simulink model "CAN_communication"  (R2022a)
settings: Solver=VariableStepAuto  StartTime=0.0  StopTime=1000.0  RelTol=1e-3
undefined symbols (not defined in the file or in its folder): canChannel
libraries: canlib x3, canmsglib x2
settings Model: Creator=Haricharan Projects  LastModifiedBy=Haricharan Projects

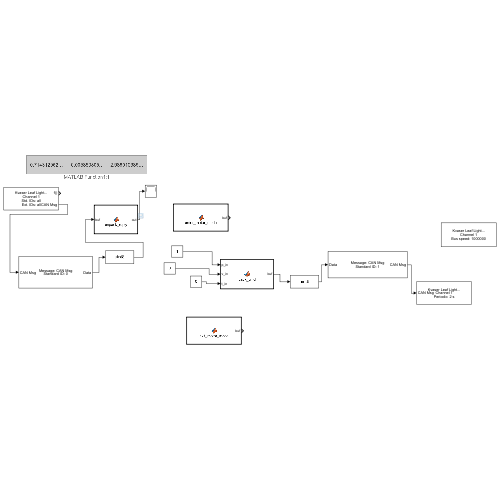
[thumbnail: Simulink's stored preview of the top-level diagram]
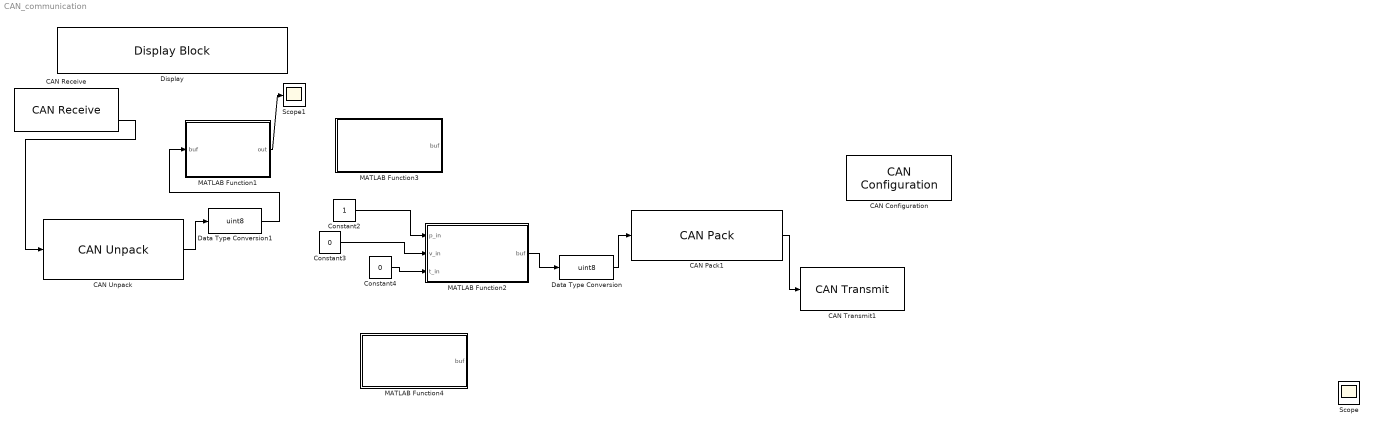
== system CAN_communication ==
  CAN Configuration : canlib/CAN Configuration  BlockHandle=12.1127  Device=MathWorks Virtual 1 (Channel 1)  DeviceMenu=MathWorks Virtual 1 (Channel 1)  ObjConstructor=canChannel('MathWorks', 'Virtual 1', 1)  BusSpeed=500000  EnableBitParameters=off  AckMode=Normal
      settings: SourceProductBaseCode=VN
  CAN Pack1 : canmsglib/CAN Pack  MsgList=(none)  MsgName=CAN Msg  MsgIDType=Standard (11-bit identifier)  MsgIdentifier=1  MsgLength=8  Remote=off  ApplyMinMax=off  BusOutput=off  SignalInfo={}
      settings: SourceProductBaseCode=XP,ME,VN  DataFormat=raw data
  CAN Receive : canlib/CAN Receive  BlockHandle=16.0028  Device=MathWorks Virtual 1 (Channel 1)  DeviceMenu=MathWorks Virtual 1 (Channel 1)  ObjConstructor=canChannel('MathWorks', 'Virtual 1', 1)  EnableStandardIDsFilter=off  StdIDsCombo=Allow all  StandardIDs=0  EnableExtendedIDsFilter=off  ExtIDsCombo=Allow all  ExtendedIDs=0  SampleTime=0.01  MsgsPerTimestep=all  InternalFilterUpdateStatus=on  BusOutput=off
      settings: SourceProductBaseCode=VN
  CAN Transmit1 : canlib/CAN Transmit  BlockHandle=19.0005  Device=MathWorks Virtual 1 (Channel 1)  DeviceMenu=MathWorks Virtual 1 (Channel 1)  ObjConstructor=canChannel('MathWorks', 'Virtual 1', 1)  EnableEventTransmit=off  EnablePeriodicTransmit=on  MessagePeriod=2.000
      settings: SourceProductBaseCode=VN
  CAN Unpack : canmsglib/CAN Unpack  MsgList=(none)  MsgName=CAN Msg  MsgIDType=Standard (11-bit identifier)  MsgIdentifier=0  MsgLength=8  SignalInfo={}  IDPort=off  TimestampPort=off  ErrorPort=off  RemotePort=off  LengthPort=off  StatusPort=off  ApplyMinMax=off
      settings: SourceProductBaseCode=XP,ME,VN  DataFormat=raw data
  Constant2 : Constant  SampleTime=2
  Constant3 : Constant  Value=0  SampleTime=2
  Constant4 : Constant  Value=0  SampleTime=2
  Data Type Conversion : DataTypeConversion  OutDataTypeStr=uint8  SaturateOnIntegerOverflow=off  RndMeth=Floor
  Data Type Conversion1 : DataTypeConversion  OutDataTypeStr=uint8  SaturateOnIntegerOverflow=off  RndMeth=Floor
  Display : DisplayBlock  LabelPosition=Bottom  Format=long  Transparency=1
  MATLAB Function1 : MATLAB Function  TreatAsAtomicUnit=on
  MATLAB Function2 : MATLAB Function  TreatAsAtomicUnit=on
  MATLAB Function3 : MATLAB Function  TreatAsAtomicUnit=on
  MATLAB Function4 : MATLAB Function  TreatAsAtomicUnit=on
  Scope1 : Scope
  Scope : Scope
  wires:
  CAN Pack1/1 -> CAN Transmit1/1
  Constant2/1 -> MATLAB Function2/1(p_in)
  Constant4/1 -> MATLAB Function2/3(t_in)
  Constant3/1 -> MATLAB Function2/2(v_in)
  CAN Receive/2 -> CAN Unpack/1
  CAN Unpack/1 -> Data Type Conversion1/1
  Data Type Conversion1/1 -> MATLAB Function1/1(buf)
  Data Type Conversion/1 -> CAN Pack1/1
  MATLAB Function1/1(out) -> Scope1/1
  MATLAB Function2/1(buf) -> Data Type Conversion/1

== matlab function CAN_communication/MATLAB Function2 ==
  data: p_in input double; buf output; v_in input; t_in input
function buf  = pack_cmd(p_in, v_in, t_in)

P_MIN = -12.5;
P_MAX = 12.5;
V_MIN = -8.0;
V_MAX = 8.0;
KP_MIN = 0.0;
KP_MAX = 500.0;
KD_MIN = 0.0;
KD_MAX = 5.0;
T_MIN = -144.0;
T_MAX = 144.0;

kp_in = 10;
kd_in = 5;

p_des = constrain(p_in, P_MIN, P_MAX);
v_des = constrain(v_in, V_MIN, V_MAX);
kp = constrain(kp_in, KP_MIN, KP_MAX);
kd = constrain(kd_in, KD_MIN, KD_MAX);
t_ff = constrain(t_in, T_MIN, T_MAX);

p_int = float_to_uint(p_des, P_MIN, P_MAX, 16);
v_int = float_to_uint(v_des, V_MIN, V_MAX, 12);
kp_int = float_to_uint(kp, KP_MIN, KP_MAX, 12);
kd_int = float_to_uint(kd, KD_MIN, KD_MAX, 12);
t_int = float_to_uint(t_ff, T_MIN, T_MAX, 12);

buf = ([0 0 0 0 0 0 0 0]);

buf(1) = bitshift(p_int, -8, 'uint64');
buf(2) = bitand(p_int, uint64(0xFF), 'uint64');
buf(3) = bitshift(v_int, -4, 'uint64');
buf(4) = bitor(bitshift(bitand(v_int, uint64(0xF), 'uint64'), +4, 'uint64'), bitshift(kp_int, -8, 'uint64'));
buf(5) = bitand(kp_int, uint64(0xFF), 'uint64');
buf(6) = bitshift(kd_int, -4, 'uint64');
buf(7) = bitor(bitshift(bitand(kd_int, uint64(0xF)), 4, 'uint64'), bitshift(t_int, -8, 'uint64'));
buf(8) = bitand(t_int, uint64(0xFF), 'uint64');

end

function [pgg] = float_to_uint(x, x_min, x_max, bits)
span = x_max - x_min;
offset = x_min;
pgg = uint64(0);

if (bits == 12)
    pgg = (x - offset) * 4095.0/ span;
    pgg = uint64(pgg);
elseif (bits == 16)
    pgg = (x - offset) * 65535.0/ span;
    pgg = uint64(pgg);
pgg = uint64(pgg);
    
end
end

function val = constrain(value, min_value, max_value)
if (value < min_value)
    val = min_value;
elseif (value > max_value)
    val = max_value;
else
    val = value;
end
end

== matlab function CAN_communication/MATLAB Function3 ==
  data: buf output
function buf = enter_motor_mode()

buf = [0 0 0 0 0 0 0 0];

buf(1) = 0xFF;
buf(2) = 0xFF;
buf(3) = 0xFF;
buf(4) = 0xFF;
buf(5) = 0xFF;
buf(6) = 0xFF;
buf(7) = 0xFF;
buf(8) = 0xFC;

end

== matlab function CAN_communication/MATLAB Function4 ==
  data: buf output
function buf = exit_motor_mode()

buf = [0 0 0 0 0 0 0 0];

buf(1) = 0xFF;
buf(2) = 0xFF;
buf(3) = 0xFF;
buf(4) = 0xFF;
buf(5) = 0xFF;
buf(6) = 0xFF;
buf(7) = 0xFF;
buf(8) = 0xFD;

end

== matlab function CAN_communication/MATLAB Function1 ==
  data: buf input; out output
function out = unpack_reply(buf)

P_MIN = -12.5;
P_MAX = 12.5;
V_MIN = -8.0;
V_MAX = 8.0;
KP_MIN = 0.0;
KP_MAX = 500.0;
KD_MIN = 0.0;
KD_MAX = 5.0;
T_MIN = -144.0;
T_MAX = 144.0;

buf = uint64(buf);

id = buf(1);
p_int = bitor(bitshift(buf(2), 8), buf(3));
v_int = bitor(bitshift(buf(4), 4), bitshift(buf(5), -4));
i_int = bitor(bitshift(bitand(buf(5), uint64(0x0F)), 8), buf(6));

p_out = uint_to_float(p_int, P_MIN, P_MAX, 16);
v_out = uint_to_float(v_int, V_MIN, V_MAX, 12);
t_out = uint_to_float(i_int, -T_MAX, T_MAX, 12);

out = [p_out v_out t_out];

end

function [pgg] = uint_to_float(x_int, x_min, x_max, bits)

span = double(x_max - x_min);
offset = double(x_min);

if (bits == 12)
    pgg = double(x_int) * span / 4095.0 + offset;
elseif (bits == 16)
    pgg = double(x_int) * span / 65535.0 + offset;
end
end
